simulink model "MotorCtrl_DTC_Math"  (R2023b)
settings: Solver=FixedStepDiscrete  StartTime=0.0  StopTime=5  FixedStep=MC_Sim_BaseStep  RelTol=1e-3  EnableMultiTasking=on
values from neighbouring files (symbols this model uses):
  MC_ADC_BitNum = 0.0    [MotorControlDataDictionary_Math.sldd]
  MC_ADC_Offset = 0.0    [MotorControlDataDictionary_Math.sldd]
  MC_ADC_VRef = 1.0    [MotorControlDataDictionary_Math.sldd]
  MC_Const_DutyL = 0.2    [MotorControlDataDictionary_Math.sldd]
  MC_Const_DutyS = 0.8    [MotorControlDataDictionary_Math.sldd]
  MC_CSA_Gain = 1.0    [MotorControlDataDictionary_Math.sldd]
  MC_Input_Vdc = 13.5    [MotorControlDataDictionary_Math.sldd]
  MC_MOS_DeadTime = 1.0E-6    [MotorControlDataDictionary_Math.sldd]
  MC_Motor_Mechinal_Damp = 1.0E-5    [MotorControlDataDictionary_Math.sldd]
  MC_Motor_Mechinal_Fric = 0.0    [MotorControlDataDictionary_Math.sldd]
  MC_Motor_Mechinal_Inertia = 0.0103    [MotorControlDataDictionary_Math.sldd]
  MC_Motor_Phi = 0.0059190254913385806    [MotorControlDataDictionary_Math.sldd]
  MC_Motor_Rotor_Pn = 4.0    [MotorControlDataDictionary_Math.sldd]
  MC_Motor_Stator_Ld = 5.6345E-5    [MotorControlDataDictionary_Math.sldd]
  MC_Motor_Stator_Lq = 5.6345E-5    [MotorControlDataDictionary_Math.sldd]
  MC_Motor_Stator_Rs = 0.0286    [MotorControlDataDictionary_Math.sldd]
  MC_Param_CurrentPI_Ki = 0.0071879639914134473    [MotorControlDataDictionary_Math.sldd]
  MC_Param_CurrentPI_Kp = 0.283220860906427    [MotorControlDataDictionary_Math.sldd]
  MC_Param_CurrentPI_UdInteMax = 7.794228634059948    [MotorControlDataDictionary_Math.sldd]
  MC_Param_CurrentPI_UdInteMin = -7.794228634059948    [MotorControlDataDictionary_Math.sldd]
  MC_Param_CurrentPI_UdMax = 7.794228634059948    [MotorControlDataDictionary_Math.sldd]
  MC_Param_CurrentPI_UdMin = -7.794228634059948    [MotorControlDataDictionary_Math.sldd]
  MC_Param_CurrentPI_UqInteMax = 7.794228634059948    [MotorControlDataDictionary_Math.sldd]
  MC_Param_CurrentPI_UqInteMin = -7.794228634059948    [MotorControlDataDictionary_Math.sldd]
  MC_Param_CurrentPI_UqMax = 7.794228634059948    [MotorControlDataDictionary_Math.sldd]
  MC_Param_CurrentPI_UqMin = -7.794228634059948    [MotorControlDataDictionary_Math.sldd]
  MC_Param_Flux_Gamma = 750000.0    [MotorControlDataDictionary_Math.sldd]
  MC_Param_Flux_Lalpha = 5.6345E-5    [MotorControlDataDictionary_Math.sldd]
  MC_Param_Flux_Lbeta = 5.6345E-5    [MotorControlDataDictionary_Math.sldd]
  MC_Param_Flux_Ralpha = 0.0286    [MotorControlDataDictionary_Math.sldd]
  MC_Param_Flux_Rbeta = 0.0286    [MotorControlDataDictionary_Math.sldd]
  MC_Param_Luen_BEMFalpha = -17747.803709290976    [MotorControlDataDictionary_Math.sldd]
  MC_Param_Luen_BEMFbeta = -17747.803709290976    [MotorControlDataDictionary_Math.sldd]
  MC_Param_Luen_BEMFErr = -8.0    [MotorControlDataDictionary_Math.sldd]
  MC_Param_Luen_Currentalpha = -507.58718608572195    [MotorControlDataDictionary_Math.sldd]
  MC_Param_Luen_Currentbeta = -507.58718608572195    [MotorControlDataDictionary_Math.sldd]
  MC_Param_Luen_CurrentErr = -8.0    [MotorControlDataDictionary_Math.sldd]
  MC_Param_Luen_PLL_Ki = 2.3480975196640594    [MotorControlDataDictionary_Math.sldd]
  MC_Param_Luen_PLL_Kp = 153.24842212633141    [MotorControlDataDictionary_Math.sldd]
  MC_Param_Luen_Voltagealpha = 17747.803709290976    [MotorControlDataDictionary_Math.sldd]
  MC_Param_Luen_Voltagebeta = 17747.803709290976    [MotorControlDataDictionary_Math.sldd]
  MC_Param_PhasetoReal = 500.0    [MotorControlDataDictionary_Math.sldd]
  MC_Param_SMO_CoffA = 0.97462064069571386    [MotorControlDataDictionary_Math.sldd]
  MC_Param_SMO_CoffB = 0.88739018546454884    [MotorControlDataDictionary_Math.sldd]
  MC_Param_SpeedCtrl_IdMax = 60.0    [MotorControlDataDictionary_Math.sldd]
  MC_Param_SpeedCtrl_IdMin = -60.0    [MotorControlDataDictionary_Math.sldd]
  MC_Param_SpeedCtrl_IqMax = 60.0    [MotorControlDataDictionary_Math.sldd]
  MC_Param_SpeedCtrl_IqMin = -60.0    [MotorControlDataDictionary_Math.sldd]
  MC_Param_SpeedPI_Ki = 0.57248683633241571    [MotorControlDataDictionary_Math.sldd]
  MC_Param_SpeedPI_Kp = 9.1114109857344836    [MotorControlDataDictionary_Math.sldd]
  MC_Param_SpeedtoTheta = 5.0E-5    [MotorControlDataDictionary_Math.sldd]
  MC_Param_SVPWM_DutyMax = 0.98    [MotorControlDataDictionary_Math.sldd]
  MC_Param_SVPWM_DutyMin = 0.02    [MotorControlDataDictionary_Math.sldd]
  MC_Param_SVPWM_SampleOffset1 = 0.02    [MotorControlDataDictionary_Math.sldd]
  MC_Param_SVPWM_SampleOffset2 = 0.015    [MotorControlDataDictionary_Math.sldd]
  MC_Param_SVPWM_SampleValid = 0.011999999999999999    [MotorControlDataDictionary_Math.sldd]
  MC_Sample_CurrentNoise = 1.0E-15    [MotorControlDataDictionary_Math.sldd]
  MC_Sample_Rs = 0.002    [MotorControlDataDictionary_Math.sldd]
  MC_Sample_VbusNoise = 1.0E-15    [MotorControlDataDictionary_Math.sldd]
  MC_Sim_BaseStep = 5.0E-8    [MotorControlDataDictionary_Math.sldd]
  MC_Sim_HFTStep = 5.0E-5    [MotorControlDataDictionary_Math.sldd]
  MC_Sim_MFTStep = 0.002    [MotorControlDataDictionary_Math.sldd]
libraries: simulink x29, spsVoltageMeasurementLib x2, spsDCVoltageSourceLib x1, spsGroundLib x1, spsPermanentMagnetSynchronousMachineLib x1, spsSeriesRLCBranchLib x1, spsThreePhaseVIMeasurementLib x1, spsUniversalBridgeLib x1, sps_lib x1
(part 3 of 5)

== system MotorCtrl_DTC_Math/Hardware_Math/MotorHardware ==
  mec : Inport
  PWM : Inport  Port=2
  DC Voltage Source : spsDCVoltageSourceLib/DC Voltage Source  Amplitude=MC_Input_Vdc  Measurements=None
  Ground : spsGroundLib/Ground  LConnTagsString=a
  Permanent Magnet Synchronous Machine1 : spsPermanentMagnetSynchronousMachineLib/Permanent Magnet Synchronous Machine  NbPhases=3  FluxDistribution=Sinusoidal  RotorType=Salient-pole  MechanicalLoad=Torque Tm  PresetModel=No  ShowDetailedParameters=on  MeasurementBus=off  Resistance=MC_Motor_Stator_Rs  Inductance=8.5e-3  dqInductances=[MC_Motor_Stator_Ld MC_Motor_Stator_Lq]  La=0.000395  MachineConstant=Voltage Constant (V_peak L-L / krpm)  Flux=0.0059185  VoltageCst=MC_Motor_BEMF  TorqueCst=0.035511  Flat=120  Mechanical=[MC_Motor_Mechinal_Inertia MC_Motor_Mechinal_Damp MC_Motor_Rotor_Pn MC_Motor_Mechinal_Fric]  PolePairs=4  InitialConditions=[0,0, 0,0]  InitialConditions5ph=[0 0 0 0 0 0]  RefAngle=Aligned with phase A axis (original Park)  IterativeDiscreteModel=Trapezoidal non iterative  TsBlock=-1  TsPowergui=0
  Series RLC Branch : spsSeriesRLCBranchLib/Series RLC Branch  LConnTagsString=__new0  RConnTagsString=__new0  BranchType=R  Resistance=MC_Sample_Rs  Inductance=1e-3  SetiL0=off  InitialCurrent=0  Capacitance=1e-6  Setx0=off  InitialVoltage=0  Measurements=None
  Three-Phase V-I Measurement : spsThreePhaseVIMeasurementLib/Three-Phase V-I Measurement  VoltageMeasurement=phase-to-ground  SetLabelV=off  LabelV=Vabc  Vpu=off  VpuLL=off  CurrentMeasurement=yes  SetLabelI=off  LabelI=Iabc  Ipu=off  Pbase=100e6  Vbase=500e3  OutputType=Complex  PhasorSimulation=off  PSBequivalent=0
  Universal Bridge : spsUniversalBridgeLib/Universal Bridge  Arms=3  SnubberResistance=1e5  SnubberCapacitance=inf  Device=MOSFET / Diodes  Ron=MC_MOS_Rds  Lon=0  ForwardVoltages="[  0  0  ]"  ForwardVoltage=MC_Hardware_MOS_Threshold  GTOparameters=[ 10e-6 , 20e-6 ]  IGBTparameters=[ 1e-6 , 2e-6 ]  Measurements=None  Measurements_2=None  converterType=Rectifier
  Voltage Measurement : spsVoltageMeasurementLib/Voltage Measurement  PhasorSimulation=off  OutputType=Complex  PSBequivalent=0
  Voltage Measurement1 : spsVoltageMeasurementLib/Voltage Measurement  PhasorSimulation=off  OutputType=Complex  PSBequivalent=0
  powergui : sps_lib/powergui  Priority=1  SimulationMode=Discrete  SampleTime=MC_Sim_BaseStep  frequency=60  Iterations=50  frequencyindice=0  Pbase=100e6  ErrMax=1e-4  UnitsV=kV  UnitsW=MW  buscounter=0  FunctionMessages=off  echomessages=off  EnableUseOfTLC=off  CurrentSourceSwitches=off  DisableSnubberDevices=off  DisableRonSwitches=off  DisableVfSwitches=off  DisplayEquations=off  AutomaticDiscreteSolvers=off  SolverType=Tustin/Backward Euler (TBE)  Interpol=off  ExternalGateDelay=off  methode=off  Ts=100  x0status=blocks  SPID=on  SwTol=0  HookPort=off  NonlinearTolerance=1e-4  nMaxIteration=100  ContinueOnMaxIteration=off  RestoreLinks=warning  ResistiveCurrentMeasurement=off  Frange=[0:2:500]  Ylog=off  Xlog=on  ShowGrid=off  save=off  variable=ZData  structure=0  ZoomFFT=off  StartTime=0.0  cycles=1  DisplayStyle=1  fundamental=60  FreqAxis=off  MaxFrequency=1000  frequencyindicesteady=1  RmsSteady=1  display=off
  Vabc : Outport
  Iabc : Outport  Port=2
  m : Outport  Port=3
  Vbus : Outport  Port=4
  Current : Outport  Port=5
  wires:
  mec/1 -> Permanent Magnet Synchronous Machine1/1
  [Vbus] -> Vbus/1  "Vbus"
  Voltage Measurement/1 -> [Vbus]
  Three-Phase V-I Measurement/1 -> Vabc/1
  Three-Phase V-I Measurement/2 -> Iabc/1
  Voltage Measurement1/1 -> Current/1  "Ibuss"
  PWM/1 -> Universal Bridge/1
  Permanent Magnet Synchronous Machine1/1 -> m/1
  connections:
  Permanent Magnet Synchronous Machine1/LConn2 -- Three-Phase V-I Measurement/RConn2
  Voltage Measurement/LConn2 -- Voltage Measurement1/LConn2 -- Series RLC Branch/RConn1 -- Ground/LConn1 -- DC Voltage Source/LConn1
  Permanent Magnet Synchronous Machine1/LConn1 -- Three-Phase V-I Measurement/RConn1
  Permanent Magnet Synchronous Machine1/LConn3 -- Three-Phase V-I Measurement/RConn3
  Universal Bridge/LConn1 -- Three-Phase V-I Measurement/LConn1
  Universal Bridge/LConn2 -- Three-Phase V-I Measurement/LConn2
  Universal Bridge/LConn3 -- Three-Phase V-I Measurement/LConn3
  Voltage Measurement1/LConn1 -- Series RLC Branch/LConn1 -- Universal Bridge/RConn2
  DC Voltage Source/RConn1 -- Universal Bridge/RConn1 -- Voltage Measurement/LConn1

== system MotorCtrl_DTC_Math/Hardware_Math/PWMGenerate ==
  DutyABC : Inport
  SamplePoint : Inport  Port=2
  Compare To Constant : simulink/Logic and Bit Operations/Compare To Constant  relop=<=  const=1  OutDataTypeStr=boolean
  Data Type Conversion{,1,3..6} (6 alike) : DataTypeConversion  SaturateOnIntegerOverflow=off  RndMeth=Floor
  Data Type Conversion2 : DataTypeConversion  OutDataTypeStr=double  SaturateOnIntegerOverflow=off  RndMeth=Floor
  DeadTimeGenerate : Subsystem
  Mux : Mux  Inputs=6
  Rate Transition : RateTransition  OutPortSampleTime=MC_Sim_BaseStep
  Rate Transition1 : RateTransition  OutPortSampleTime=MC_Sim_BaseStep
  Relational Operator{,2..3,5} (4 alike) : RelationalOperator  OutDataTypeStr=boolean  RndMeth=Simplest  InputSameDT=off
  Relational Operator1 : RelationalOperator  Operator=<=  OutDataTypeStr=boolean  RndMeth=Simplest  InputSameDT=off
  Relational Operator4 : RelationalOperator  Operator=<=  OutDataTypeStr=boolean  RndMeth=Simplest  InputSameDT=off
  Relational Operator6 : RelationalOperator  Operator=<=  OutDataTypeStr=boolean  RndMeth=Simplest  InputSameDT=off
  Repeating Sequence : simulink/Sources/Repeating Sequence  rep_seq_t=[0 MC_Sim_HFTStep/2 MC_Sim_HFTStep]  rep_seq_y=[0 1 2]
  Repeating Sequence1 : simulink/Sources/Repeating Sequence  rep_seq_t=[0 MC_Sim_HFTStep/2 MC_Sim_HFTStep]  rep_seq_y=[2 1 0]
  Switch : Switch  Criteria=u2 > Threshold  SaturateOnIntegerOverflow=off  InputSameDT=off
  Gate : Outport
  CurrentSamplTrigger : Outport  Port=2
  wires:
  Data Type Conversion6/1 -> Mux/6  "PWMCDOWN"
  Data Type Conversion5/1 -> Mux/5  "PWMCUP"
  Data Type Conversion4/1 -> Mux/4  "PWMBDOWN"
  Data Type Conversion3/1 -> Mux/3  "PWMBUP"
  Data Type Conversion1/1 -> Mux/2  "PWMADOWN"
  Data Type Conversion/1 -> Mux/1  "PWMAUP"
  DeadTimeGenerate/6(GateCL) -> Relational Operator6/2
  DeadTimeGenerate/5(GateCH) -> Relational Operator5/2
  DeadTimeGenerate/4(GateBL) -> Relational Operator4/2
  DeadTimeGenerate/3(GateBH) -> Relational Operator2/2
  Relational Operator6/1 -> Data Type Conversion6/1
  Relational Operator5/1 -> Data Type Conversion5/1
  Relational Operator4/1 -> Data Type Conversion4/1
  Relational Operator2/1 -> Data Type Conversion3/1
  Relational Operator1/1 -> Data Type Conversion1/1
  Relational Operator/1 -> Data Type Conversion/1
  Repeating Sequence/1 -> Switch/1, Compare To Constant/1
  Repeating Sequence1/1 -> Switch/3
  DutyABC/1 -> DeadTimeGenerate/2(DutyABC)
  DeadTimeGenerate/1(GateAH) -> Relational Operator/2
  Switch/1 -> Rate Transition/1
  DeadTimeGenerate/2(GateAL) -> Relational Operator1/2
  Relational Operator3/1 -> Data Type Conversion2/1
  SamplePoint/1 -> Relational Operator3/2
  Data Type Conversion2/1 -> CurrentSamplTrigger/1  "CurrentSamplTrigger"
  Compare To Constant/1 -> Rate Transition1/1
  Mux/1 -> Gate/1  "Gate"
  Rate Transition/1 -> Relational Operator/1, Relational Operator1/1, Relational Operator3/1, Relational Operator6/1, Relational Operator5/1, Relational Operator4/1, Relational Operator2/1
  Rate Transition1/1 -> DeadTimeGenerate/1(FLag), Switch/2

== system MotorCtrl_DTC_Math/Hardware_Math/VbusSample ==
  Vbus : Inport
  ADCOffset : Constant  Value=0  SampleTime=-1
  ADCQuality : Gain
  Add : Sum
  Data Type Conversion3 : DataTypeConversion  OutDataTypeStr=single  SaturateOnIntegerOverflow=off  RndMeth=Floor
  VbusSample : Outport
  wires:
  Vbus/1 -> Add/2
  Add/1 -> ADCQuality/1
  ADCQuality/1 -> Data Type Conversion3/1
  ADCOffset/1 -> Add/1
  Data Type Conversion3/1 -> VbusSample/1  "PhaseI"

== system MotorCtrl_DTC_Math/Hardware_Math/currentSample ==
  SampleTrigger : Inport
  Current : Inport  Port=2
  getCurrentSample_ORS_Double : Subsystem  VariantControl=MC_Sample_Model==1 && MC_Sample_ORSType == 2
  getCurrentSample_ORS_Single : Subsystem  VariantControl=MC_Sample_Model==1 && MC_Sample_ORSType == 1
  getCurrentSample_TRS(Three) : Subsystem  VariantControl=MC_Sample_Model==3
  getCurrentSample_TRS(Two) : Subsystem  VariantControl=MC_Sample_Model==2
  SampleCurrent : Outport

== system MotorCtrl_DTC_Math/MFTask/getCurrentLimit ==
  IdRef : Inport
  IqRef : Inport  Port=2
  Saturation : Saturate  UpperLimit=MC_Param_SpeedCtrl_IqMax  LowerLimit=MC_Param_SpeedCtrl_IqMin
  Saturation1 : Saturate  UpperLimit=MC_Param_SpeedCtrl_IdMax  LowerLimit=MC_Param_SpeedCtrl_IdMin
  Signal Copy : SignalConversion  OverrideOpt=off
  Signal Copy1 : SignalConversion  OverrideOpt=off
  IdRefLimit : Outport
  IqRefLimit : Outport  Port=2
  wires:
  IqRef/1 -> Saturation/1
  IdRef/1 -> Saturation1/1
  Signal Copy/1 -> IdRefLimit/1  "IdRefLimit"
  Signal Copy1/1 -> IqRefLimit/1  "IqRefLimit"
  Saturation/1 -> Signal Copy1/1
  Saturation1/1 -> Signal Copy/1

== system MotorCtrl_DTC_Math/MFTask/piofSpeed ==
  SpeedTarget : Inport
  SpeedReal : Inport  Port=2
  Abs : Abs  SaturateOnIntegerOverflow=off
  Add : Sum
  Add1 : Sum
  Compare To Constant : simulink/Logic and Bit Operations/Compare To Constant  relop=>  const=0.01  OutDataTypeStr=boolean
  Constant : Constant  Value=0  OutDataTypeStr=single
  Constant1 : Constant  Value=0  OutDataTypeStr=single
  Delay One Step : Delay  DelayLength=1
  Gain : Gain  Gain=MC_Param_SpeedPI_Kp
  Gain1 : Gain  Gain=MC_Param_SpeedPI_Ki
  Saturation : Saturate  UpperLimit=50  LowerLimit=-50
  Saturation1 : Saturate  UpperLimit=100  LowerLimit=-100
  Subtract : Sum  Inputs=+-
  Switch : Switch  Criteria=u2 > Threshold  SaturateOnIntegerOverflow=off  InputSameDT=off
  IdRef : Outport
  IqRef : Outport  Port=2
  wires:
  Add/1 -> Saturation/1, Delay One Step/1
  Subtract/1 -> Switch/1, Abs/1, Gain/1
  Gain1/1 -> Add/1
  Saturation/1 -> Add1/2
  Delay One Step/1 -> Add/2
  Gain/1 -> Add1/1
  Compare To Constant/1 -> Switch/2
  Add1/1 -> Saturation1/1
  Abs/1 -> Compare To Constant/1
  Constant/1 -> Switch/3
  SpeedReal/1 -> Subtract/2
  SpeedTarget/1 -> Subtract/1
  Switch/1 -> Gain1/1
  Constant1/1 -> IdRef/1  "IdRef"
  Saturation1/1 -> IqRef/1  "IqRef"

== system MotorCtrl_DTC_Math/MFTask/smcofSpeed ==
  SpeedTarget : Inport
  SpeedReal : Inport  Port=2
  Add : Sum
  Add1 : Sum
  Add2 : Sum
  Constant : Constant  Value=0  OutDataTypeStr=single
  Delay One Step : Delay  DelayLength=1
  Delay One Step1 : Delay  DelayLength=1
  Gain : Gain  Gain=1/MC_Sim_MFTStep
  Gain1 : Gain  Gain=200
  Gain2 : Gain  Gain=50
  Gain3 : Gain  Gain=MC_Sim_MFTStep*1*MC_Motor_Mechinal_Inertia/(3*MC_Motor_Phi*MC_Motor_Rotor_Pn)
  Saturation : Saturate  UpperLimit=2  LowerLimit=-2
  Subtract : Sum  Inputs=+-
  Subtract1 : Sum  Inputs=+-
  IdRef : Outport
  IqRef : Outport  Port=2
  wires:
  SpeedTarget/1 -> Subtract/1
  SpeedReal/1 -> Subtract/2
  Subtract/1 -> Delay One Step/1, Subtract1/1, Add/1  "E1"
  Delay One Step/1 -> Subtract1/2
  Subtract1/1 -> Gain/1
  Gain/1 -> Add/2, Gain2/1  "E2"
  Add/1 -> Saturation/1  "S"
  Saturation/1 -> Gain1/1  "sign(S)"
  Gain1/1 -> Add1/1
  Gain2/1 -> Add1/2
  Add1/1 -> Gain3/1  "IqRef_dot"
  Gain3/1 -> Add2/1
  Add2/1 -> IqRef/1, Delay One Step1/1  "IqRef"
  Delay One Step1/1 -> Add2/2
  Constant/1 -> IdRef/1  "IdRef"

== system MotorCtrl_DTC_Math/svpwm_OM/getVoltageExchange ==
  Valpha : Inport
  Vbeta : Inport  Port=2
  Vdc : Inport  Port=3
  Add : Sum
  Add1 : Sum
  Divide : Product  Inputs=*/
  Divide1 : Product  Inputs=*/
  Gain : Gain  Gain=-1/2
  Gain1 : Gain  Gain=sqrt(3)/2
  Gain2 : Gain  Gain=-1
  Relational Operator : RelationalOperator  OutDataTypeStr=boolean  RndMeth=Simplest  InputSameDT=off
  Relational Operator1 : RelationalOperator  OutDataTypeStr=boolean  RndMeth=Simplest  InputSameDT=off
  Relational Operator2 : RelationalOperator  Operator=<=  OutDataTypeStr=boolean  RndMeth=Simplest  InputSameDT=off
  Relational Operator3 : RelationalOperator  Operator=<=  OutDataTypeStr=boolean  RndMeth=Simplest  InputSameDT=off
  Signal Copy : SignalConversion  OverrideOpt=off
  Subtract : Sum  Inputs=+-
  Switch{,1..3} (4 alike) : Switch  Criteria=u2 > Threshold  SaturateOnIntegerOverflow=off  InputSameDT=off
  getSectorN : Subsystem  Commented=on
  Va : Outport
  Vb : Outport  Port=2
  Vc : Outport  Port=3
  Vmed : Outport  Port=4
  wires:
  Gain2/1 -> Vmed/1  "Vmed"
  Add1/1 -> Gain2/1
  Relational Operator2/1 -> Switch2/2
  Switch2/1 -> Relational Operator3/1, Switch3/1
  Relational Operator3/1 -> Switch3/2
  Switch3/1 -> Add1/2  "Vmin"
  Relational Operator/1 -> Switch/2
  Switch/1 -> Switch1/1, Relational Operator1/1
  Relational Operator1/1 -> Switch1/2
  Switch1/1 -> Add1/1  "Vmax"
  Signal Copy/1 -> Va/1, Relational Operator/1, Switch/1, Relational Operator2/1, Switch2/1  "Va"
  Divide/1 -> Signal Copy/1, Gain/1
  Divide1/1 -> Gain1/1
  Gain/1 -> Subtract/1, Add/1
  Gain1/1 -> Add/2, Subtract/2
  Add/1 -> Vb/1, Relational Operator/2, Switch/3, Relational Operator2/2, Switch2/3  "Vb"
  Subtract/1 -> Vc/1, Switch1/3, Relational Operator1/2, Switch3/3, Relational Operator3/2  "Vc"
  Vdc/1 -> Divide1/2, Divide/2
  Vbeta/1 -> Divide1/1
  Valpha/1 -> Divide/1

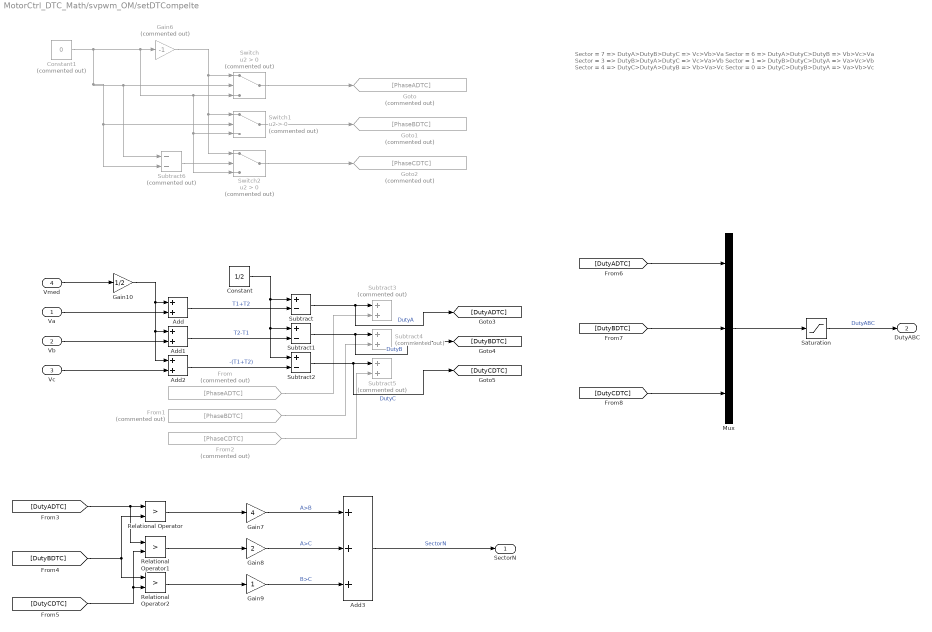
== system MotorCtrl_DTC_Math/svpwm_OM/setDTCompelte ==
  note: Sector = 7 => DutyA>DutyB>DutyC => Vc>Vb>Va
      | Sector = 6 => DutyA>DutyC>DutyB => Vb>Vc>Va
      | Sector = 3 => DutyB>DutyA>DutyC => Vc>Va>Vb
      | Sector = 1 => DutyB>DutyC>DutyA => Va>Vc>Vb
      | Sector = 4 => DutyC>DutyA>DutyB => Vb>Va>Vc
      | Sector = 0 => DutyC>DutyB>DutyA => Va>Vb>Vc
  Va : Inport
  Vb : Inport  Port=2
  Vc : Inport  Port=3
  Vmed : Inport  Port=4
  Add : Sum
  Add1 : Sum
  Add2 : Sum
  Add3 : Sum  Inputs=+++
  Constant : Constant  Value=1/2  OutDataTypeStr=single
  Constant1 : Constant  Commented=on  Value=0  OutDataTypeStr=single
  From : From  Commented=on  GotoTag=PhaseADTC
  From1 : From  Commented=on  GotoTag=PhaseBDTC
  From2 : From  Commented=on  GotoTag=PhaseCDTC
  Gain10 : Gain  Gain=1/2
  Gain6 : Gain  Commented=on  Gain=-1
  Gain7 : Gain  Gain=4  OutDataTypeStr=single  RndMeth=Simplest
  Gain8 : Gain  Gain=2  OutDataTypeStr=single  RndMeth=Simplest
  Gain9 : Gain  OutDataTypeStr=single  RndMeth=Simplest
  Goto : Goto  Commented=on  GotoTag=PhaseADTC
  Goto1 : Goto  Commented=on  GotoTag=PhaseBDTC
  Goto2 : Goto  Commented=on  GotoTag=PhaseCDTC
  Mux : Mux  Inputs=3
  Relational Operator : RelationalOperator  Operator=>  OutDataTypeStr=boolean  RndMeth=Simplest  InputSameDT=off
  Relational Operator1 : RelationalOperator  Operator=>  OutDataTypeStr=boolean  RndMeth=Simplest  InputSameDT=off
  Relational Operator2 : RelationalOperator  Operator=>  OutDataTypeStr=boolean  RndMeth=Simplest  InputSameDT=off
  Saturation : Saturate  UpperLimit=MC_Param_SVPWM_DutyMax  LowerLimit=MC_Param_SVPWM_DutyMin
      settings: AttributesFormatString=|
      | OutputMax = %<UpperLimit>
      | OutputMin = %<LowerLimit>
  Subtract : Sum  Inputs=+-
  Subtract1 : Sum  Inputs=+-
  Subtract2 : Sum  Inputs=+-
  Subtract3 : Sum  Commented=on
  Subtract4 : Sum  Commented=on
  Subtract5 : Sum  Commented=on
  Subtract6 : Sum  Commented=on  Inputs=--
  Switch : Switch  Commented=on  Criteria=u2 > Threshold  SaturateOnIntegerOverflow=off  InputSameDT=off
  Switch1 : Switch  Commented=on  Criteria=u2 > Threshold  SaturateOnIntegerOverflow=off  InputSameDT=off
  Switch2 : Switch  Commented=on  Criteria=u2 > Threshold  SaturateOnIntegerOverflow=off  InputSameDT=off
  SectorN : Outport
  DutyABC : Outport  Port=2
  wires:
  Saturation/1 -> DutyABC/1  "DutyABC"
  Mux/1 -> Saturation/1
  Gain10/1 -> Add/1, Add1/1, Add2/1
  Add3/1 -> SectorN/1  "SectorN"
  Gain7/1 -> Add3/1  "A>B"
  Gain9/1 -> Add3/3  "B>C"
  Gain8/1 -> Add3/2  "A>C"
  Relational Operator2/1 -> Gain9/1
  Relational Operator1/1 -> Gain8/1
  Relational Operator/1 -> Gain7/1
  [DutyCDTC] -> Relational Operator1/2, Relational Operator2/2
  [DutyADTC] -> Relational Operator/1, Relational Operator1/1
  [DutyBDTC] -> Relational Operator2/1, Relational Operator/2
  From2/1 -> Subtract5/2
  From1/1 -> Subtract4/2
  From/1 -> Subtract3/2
  Switch2/1 -> Goto2/1
  Switch1/1 -> Goto1/1
  Switch/1 -> Goto/1
  Subtract6/1 -> Switch2/2
  Constant1/1 -> Switch1/2, Subtract6/2, Switch/2, Subtract6/1, Gain6/1, Switch/3, Switch1/3, Switch2/3
  Gain6/1 -> Switch/1, Switch1/1, Switch2/1
  Subtract2/1 -> [DutyCDTC], Subtract5/1  "DutyC"
  Subtract1/1 -> [DutyBDTC], Subtract4/1  "DutyB"
  Subtract/1 -> [DutyADTC], Subtract3/1  "DutyA"
  Constant/1 -> Subtract/1, Subtract1/1, Subtract2/1
  Add1/1 -> Subtract1/2  "T2-T1"
  Add2/1 -> Subtract2/2  "-(T1+T2)"
  Add/1 -> Subtract/2  "T1+T2"
  Vc/1 -> Add2/2
  Vb/1 -> Add1/2
  Vmed/1 -> Gain10/1
  Va/1 -> Add/2
  [DutyADTC] -> Mux/1
  [DutyBDTC] -> Mux/2
  [DutyCDTC] -> Mux/3

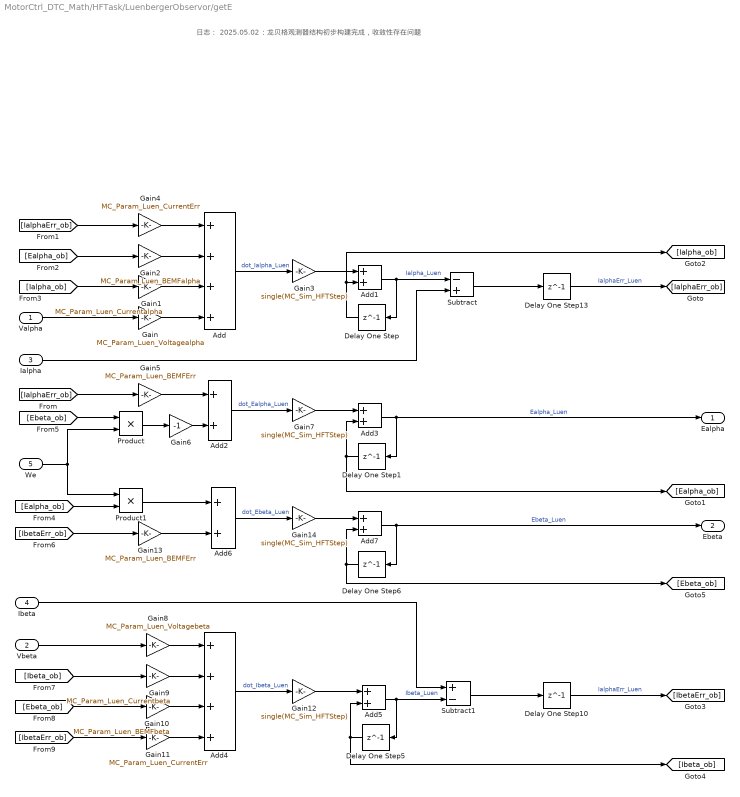
== system MotorCtrl_DTC_Math/HFTask/LuenbergerObservor/getE ==
  note: 日志：
      | 2025.05.02：龙贝格观测器结构初步构建完成，收敛性存在问题
  Valpha : Inport
  Vbeta : Inport  Port=2
  Ialpha : Inport  Port=3
  Ibeta : Inport  Port=4
  We : Inport  Port=5
  Add : Sum  Inputs=++++
  Add{1..3,5..7} (6 alike) : Sum
  Add4 : Sum  Inputs=++++
  Delay One Step{,1,5..6,10,13} (6 alike) : Delay  DelayLength=1
  Gain : Gain  Gain=MC_Param_Luen_Voltagealpha
  Gain1 : Gain  Gain=MC_Param_Luen_Currentalpha
  Gain10 : Gain  Gain=MC_Param_Luen_BEMFbeta
  Gain11 : Gain  Gain=MC_Param_Luen_CurrentErr
  Gain{3,7,12,14} (4 alike) : Gain  Gain=single(MC_Sim_HFTStep)
  Gain13 : Gain  Gain=MC_Param_Luen_BEMFErr
  Gain2 : Gain  Gain=MC_Param_Luen_BEMFalpha
  Gain4 : Gain  Gain=MC_Param_Luen_CurrentErr
  Gain5 : Gain  Gain=MC_Param_Luen_BEMFErr
  Gain6 : Gain  Gain=-1
  Gain8 : Gain  Gain=MC_Param_Luen_Voltagebeta
  Gain9 : Gain  Gain=MC_Param_Luen_Currentbeta
  Product : Product
  Product1 : Product
  Subtract : Sum  Inputs=-+
  Subtract1 : Sum  Inputs=+-
  Ealpha : Outport
  Ebeta : Outport  Port=2
  wires:
  Valpha/1 -> Gain/1
  Add/1 -> Gain3/1  "dot_Ialpha_Luen"
  Gain2/1 -> Add/2
  Gain1/1 -> Add/3
  Gain/1 -> Add/4
  Gain4/1 -> Add/1
  Gain3/1 -> Add1/1
  Add1/1 -> Subtract/1, Delay One Step/1  "Ialpha_Luen"
  Delay One Step/1 -> [Ialpha_ob], Add1/2
  Ialpha/1 -> Subtract/2
  Subtract/1 -> Delay One Step13/1
  [IalphaErr_ob] -> Gain5/1
  Gain5/1 -> Add2/1
  Gain6/1 -> Add2/2
  Add2/1 -> Gain7/1  "dot_Ealpha_Luen"
  Delay One Step1/1 -> Add3/2, [Ealpha_ob]
  Add3/1 -> Ealpha/1, Delay One Step1/1  "Ealpha_Luen"
  Gain7/1 -> Add3/1
  Product/1 -> Gain6/1
  We/1 -> Product/2, Product1/1
  Vbeta/1 -> Gain8/1
  Gain8/1 -> Add4/1
  Gain9/1 -> Add4/2
  Gain10/1 -> Add4/3
  Gain11/1 -> Add4/4
  [IalphaErr_ob] -> Gain4/1
  [Ealpha_ob] -> Gain2/1
  [Ialpha_ob] -> Gain1/1
  Add4/1 -> Gain12/1  "dot_Ibeta_Luen"
  Delay One Step5/1 -> Add5/2, [Ibeta_ob]
  Add5/1 -> Subtract1/2, Delay One Step5/1  "Ibeta_Luen"
  Gain12/1 -> Add5/1
  Ibeta/1 -> Subtract1/1
  Subtract1/1 -> Delay One Step10/1
  Add6/1 -> Gain14/1  "dot_Ebeta_Luen"
  Gain13/1 -> Add6/2
  Product1/1 -> Add6/1
  Gain14/1 -> Add7/1
  Add7/1 -> Ebeta/1, Delay One Step6/1  "Ebeta_Luen"
  Delay One Step6/1 -> Add7/2, [Ebeta_ob]
  [Ealpha_ob] -> Product1/2
  [Ebeta_ob] -> Product/1
  [IbetaErr_ob] -> Gain13/1
  [Ibeta_ob] -> Gain9/1
  [IbetaErr_ob] -> Gain11/1
  [Ebeta_ob] -> Gain10/1
  Delay One Step13/1 -> [IalphaErr_ob]  "IalphaErr_Luen"
  Delay One Step10/1 -> [IbetaErr_ob]  "IalphaErr_Luen"

== system MotorCtrl_DTC_Math/HFTask/LuenbergerObservor/getSpeedandTheta ==
  note: 日志：
      | 2025.03.19：反电势正负号识别错误，改正后可以使用
  Ealpha : Inport
  Ebeta : Inport  Port=2
  Add : Sum
  Add1 : Sum
  Add2 : Sum
  Constant : Constant  Value=2*pi  OutDataTypeStr=single
  Delay One Step : Delay  DelayLength=1
  Delay One Step2 : Delay  DelayLength=1
  Gain1 : Gain  Gain=MC_Param_Luen_PLL_Kp
  Gain2 : Gain  Gain=MC_Param_Luen_PLL_Ki
  Gain3 : Gain  Gain=MC_Param_SpeedtoTheta
  Gain5 : Gain  Gain=30/(pi*MC_Motor_Rotor_Pn)  OutDataTypeStr=single  RndMeth=Simplest
  Mod : Math  Operator=mod
  Product : Product
  Product1 : Product
  Sin : Trigonometry  OutputSignalType=real
  Sin1 : Trigonometry  Operator=cos  OutputSignalType=real
  Subtract : Sum  Inputs=+-
  Speed : Outport
  Theta : Outport  Port=2
  We : Outport  Port=3
  wires:
  Gain5/1 -> Speed/1  "SpeedLuen_RPM"
  Product1/1 -> Subtract/2  "LuenCos"
  Product/1 -> Subtract/1  "LuenSin"
  [Theta_Last] -> Sin/1, Sin1/1
  Add1/1 -> We/1, Gain3/1, Gain5/1  "WeLuen"
  Mod/1 -> Delay One Step2/1, Theta/1  "ThetaLuen"
  Delay One Step2/1 -> [Theta_Last], Add2/2
  Constant/1 -> Mod/2
  Add2/1 -> Mod/1
  Gain3/1 -> Add2/1
  Subtract/1 -> Gain1/1, Gain2/1  "LuenErr"
  Gain1/1 -> Add1/1
  Delay One Step/1 -> Add/2
  Add/1 -> Add1/2, Delay One Step/1
  Gain2/1 -> Add/1
  Sin/1 -> Product1/2
  Sin1/1 -> Product/2
  Ealpha/1 -> Product1/1
  Ebeta/1 -> Product/1

== system MotorCtrl_DTC_Math/HFTask/fluxobservor/getFlux ==
  note: 日志：
      | 2025.02.28：滑膜观测器建模无问题，但是反电势观测存在问题，暂时分析为参数问题
  Valpha : Inport
  Vbeta : Inport  Port=2
  Ialpha : Inport  Port=3
  Ibeta : Inport  Port=4
  Add{,1..4} (5 alike) : Sum
  Constant : Constant  Value=MC_Motor_Phi  OutDataTypeStr=single
  Delay One Step{,1..3} (4 alike) : Delay  DelayLength=1
  Gain : Gain  Gain=MC_Param_Flux_Ralpha
  Gain1 : Gain  Gain=MC_Param_Flux_Gamma  OutDataTypeStr=single  RndMeth=Simplest
  Gain2 : Gain  Gain=single(MC_Sim_HFTStep)  OutDataTypeStr=single  RndMeth=Simplest
  Gain3 : Gain  Gain=MC_Param_Flux_Lalpha  OutDataTypeStr=single  RndMeth=Simplest
  Gain4 : Gain  Gain=MC_Param_Flux_Rbeta
  Gain5 : Gain  Gain=MC_Param_Flux_Gamma  OutDataTypeStr=single  RndMeth=Simplest
  Gain6 : Gain  Gain=single(MC_Sim_HFTStep)
  Gain7 : Gain  Gain=MC_Param_Flux_Lbeta  OutDataTypeStr=single  RndMeth=Simplest
  Product : Product
  Product1 : Product
  Square : Math  Operator=square
  Square1 : Math  Operator=square
  Square2 : Math  Operator=square
  Subtract{,1..4} (5 alike) : Sum  Inputs=+-
  Phialpha : Outport
  Phibeta : Outport  Port=2
  wires:
  Valpha/1 -> Subtract/1
  Ialpha/1 -> Gain3/1, Gain/1
  Gain/1 -> Subtract/2
  Subtract/1 -> Add/1
  Gain1/1 -> Add/2
  Add/1 -> Gain2/1
  Add1/1 -> Subtract1/1, Delay One Step/1
  Delay One Step/1 -> Add1/2
  Gain2/1 -> Add1/1
  Gain3/1 -> Subtract1/2
  Subtract1/1 -> Phialpha/1, Delay One Step1/1  "Phialpha"
  Product/1 -> Gain1/1
  Delay One Step1/1 -> [Nx_alpha], Product/2
  Delay One Step3/1 -> [Nx_beta], Product1/2
  Product1/1 -> Gain5/1
  Subtract3/1 -> Phibeta/1, Delay One Step3/1  "Phibeta"
  Gain7/1 -> Subtract3/2
  Gain6/1 -> Add3/1
  Delay One Step2/1 -> Add3/2
  Add3/1 -> Delay One Step2/1, Subtract3/1
  Add2/1 -> Gain6/1
  Gain5/1 -> Add2/2
  Subtract2/1 -> Add2/1
  Gain4/1 -> Subtract2/2
  Ibeta/1 -> Gain4/1, Gain7/1
  Vbeta/1 -> Subtract2/1
  Constant/1 -> Square/1
  [Nx_alpha] -> Square1/1
  [Nx_beta] -> Square2/1
  Square1/1 -> Add4/1
  Square2/1 -> Add4/2
  Square/1 -> Subtract4/1
  Add4/1 -> Subtract4/2
  Subtract4/1 -> [Nx2]
  [Nx2] -> Product/1
  [Nx2] -> Product1/1

== system MotorCtrl_DTC_Math/HFTask/fluxobservor/getSpeedandTheta ==
  Phialpha : Inport
  Phibeta : Inport  Port=2
  Add : Sum
  Add1 : Sum
  Add2 : Sum
  Constant : Constant  Value=2*pi  OutDataTypeStr=single
  Delay One Step : Delay  DelayLength=1
  Delay One Step2 : Delay  DelayLength=1
  Gain : Gain  Gain=1/MC_Motor_Phi
  Gain1 : Gain  Gain=2*sqrt(2)/2*100
  Gain2 : Gain  Gain=100^2*MC_Sim_HFTStep
  Gain3 : Gain  Gain=MC_Param_SpeedtoTheta  OutDataTypeStr=single  RndMeth=Simplest
  Gain4 : Gain  Gain=1/MC_Motor_Phi
  Gain5 : Gain  Gain=30/(pi*MC_Motor_Rotor_Pn)  OutDataTypeStr=single  RndMeth=Simplest
  Mod : Math  Operator=mod
  Product : Product
  Product1 : Product
  Sin : Trigonometry  OutputSignalType=real
  Sin1 : Trigonometry  Operator=cos  OutputSignalType=real
  Subtract : Sum  Inputs=+-
  Speed : Outport
  Theta : Outport  Port=2
  wires:
  [Theta_Last] -> Sin/1, Sin1/1
  Add1/1 -> Gain5/1, Gain3/1  "WeFlux"
  Mod/1 -> Delay One Step2/1, Theta/1  "ThetaFlux"
  Delay One Step2/1 -> [Theta_Last], Add2/2
  Constant/1 -> Mod/2
  Add2/1 -> Mod/1
  Gain3/1 -> Add2/1
  Subtract/1 -> Gain1/1, Gain2/1  "FluxErr"
  Gain1/1 -> Add1/1
  Delay One Step/1 -> Add/2
  Add/1 -> Add1/2, Delay One Step/1
  Gain2/1 -> Add/1
  Product1/1 -> Subtract/2  "FluxSin"
  Product/1 -> Subtract/1  "FluxCos"
  Sin/1 -> Product1/2
  Sin1/1 -> Product/2
  Phibeta/1 -> Gain/1
  Phialpha/1 -> Gain4/1
  Gain/1 -> Product/1
  Gain4/1 -> Product1/1
  Gain5/1 -> Speed/1  "SpeedFlux_RPM"

== system MotorCtrl_DTC_Math/HFTask/smo/getE ==
  note: 日志：
      | 2025.02.28：滑膜观测器建模无问题，但是反电势观测存在问题，暂时分析为参数问题
  Valpha : Inport
  Vbeta : Inport  Port=2
  Ialpha : Inport  Port=3
  Ibeta : Inport  Port=4
  Add : Sum  Inputs=--+
  Add1 : Sum
  Add2 : Sum  Inputs=+--
  Add3 : Sum
  Delay One Step{,1..3} (4 alike) : Delay  DelayLength=1
  Gain{,4,6,8} (4 alike) : Gain  Gain=MC_Param_SMO_CoffB
  Gain3 : Gain  Gain=MC_Param_SMO_CoffA
  Gain7 : Gain  Gain=MC_Param_SMO_CoffA
  Saturation : Saturate  UpperLimit=100  LowerLimit=-100
  Saturation1 : Saturate  UpperLimit=100  LowerLimit=-100
  Subtract : Sum  Inputs=+-
  Subtract1 : Sum  Inputs=-+
  Ealpha : Outport
  Ebeta : Outport  Port=2
  wires:
  Valpha/1 -> Gain/1
  Add1/1 -> Subtract/1, Delay One Step/1  "Ialpha_Ob"
  Ialpha/1 -> Subtract/2
  Gain/1 -> Add/3
  Gain3/1 -> Add/2
  Gain4/1 -> Add/1
  Delay One Step1/1 -> [Ealpha_SMO]
  [Ialpha_SMO] -> Gain3/1
  [Ealpha_SMO] -> Gain4/1
  Subtract/1 -> Saturation/1  "Ialpha_ob-Ialpha"
  Saturation/1 -> Ealpha/1, Delay One Step1/1  "Ealpha"
  Gain6/1 -> Add2/1
  Gain7/1 -> Add2/2
  Gain8/1 -> Add2/3
  Vbeta/1 -> Gain6/1
  Add/1 -> Add1/1  "dotIalpha_ob"
  Delay One Step/1 -> Add1/2, [Ialpha_SMO]
  Add2/1 -> Add3/2  "dotIbeta_ob"
  Add3/1 -> Subtract1/2, Delay One Step2/1  "Ibeta_Ob"
  Delay One Step2/1 -> [Ibeta_SMO], Add3/1
  Ibeta/1 -> Subtract1/1
  Subtract1/1 -> Saturation1/1  "Ibeta_ob-Ibeta"
  Saturation1/1 -> Ebeta/1, Delay One Step3/1  "Ebeta"
  Delay One Step3/1 -> [Ebeta_SMO]
  [Ibeta_SMO] -> Gain7/1
  [Ebeta_SMO] -> Gain8/1
